simulink model "MagnetoShield_PolePlacement_UNO"  (R2019a)
settings: Solver=FixedStepAuto  StartTime=0.0  StopTime=10.0  RelTol=1e-3  EnableMultiTasking=on
undefined symbols (not defined in the file): A, B, C, DiscIntNeverNeededParam, i0, K, L, MEGA, Ts, u0, UNO, y0
libraries: MagnetoLibrary x2, CommonBlocks x1
settings Model: SimulationMode=external  ExtModeTrigDuration=2  Creator=jakub  LastModifiedBy=jakub
settings OptimizationCC: EnhancedBackFolding=on  PassReuseOutputArgsAs=Individual arguments  MaxStackSize=64  OptimizeBlockOrder=speed  DifferentSizesBufferReuse=on  OptimizationCustomize=off
settings DebuggingCC: ParameterTunabilityLossMsg=error
settings HardwareCC: ProdBitPerInt=16  ProdBitPerPointer=16  ProdBitPerSizeT=16  ProdBitPerPtrDiffT=16  ProdLargestAtomicFloat=None  ProdWordSize=8  ProdHWDeviceType=Atmel->AVR
settings SFSimCC: MATLABDynamicMemAlloc=off
settings RTWCC: SystemTargetFile=ert.tlc  HardwareBoard=Arduino Uno  TLCOptions=-aInlineSetEventsForThisBaseRateFcn=TLC_FALSE -aSuppressMultiTaskScheduler=TLC_FALSE -aRateBasedStepFcn=1  TemplateMakefile=ert_default_tmf  GenerateReport=on  Toolchain=Arduino AVR  BuildConfiguration=Faster Runs  IncludeHyperlinkInReport=on  LaunchReport=on  GenerateTraceInfo=on  GenerateTraceReport=on  GenerateTraceReportSl=on  GenerateTraceReportSf=on  GenerateTraceReportEml=on
settings CodeAppCC: ForceParamTrailComments=on  IgnoreCustomStorageClasses=off  OperatorAnnotations=on  SimulinkDataObjDesc=on  SFDataObjDesc=on  InsertBlockDesc=on
settings ERTTargetCC: SupportContinuousTime=on  SupportVariableSizeSignals=on  ExtModeStaticAllocSize=250

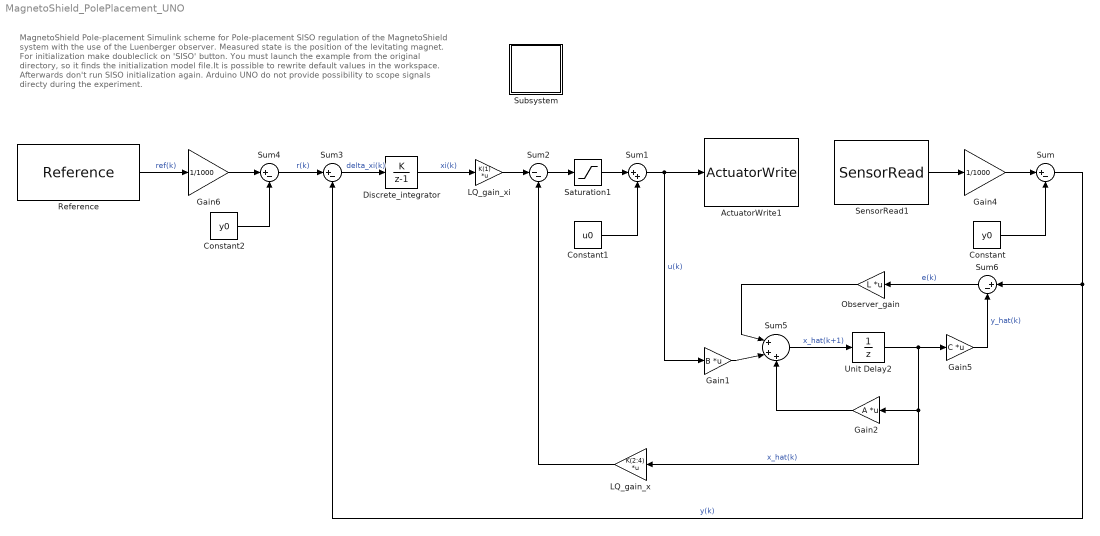
== system MagnetoShield_PolePlacement_UNO ==
  note: MagnetoShield Pole-placement
      | Simulink scheme for Pole-placement SISO regulation of the MagnetoShield system with the use of the Luenberger
      | observer. Measured state is the position of the levitating magnet.
      | For initialization make doubleclick on 'SISO' button. You must launch the example from the original directory, so it
      | finds the initialization model file.It is possible to rewrite default values in the workspace. Afterwards don't run SISO
      | initialization again.
      | Arduino UNO do not provide possibility to scope signals directy during the experiment.
  ActuatorWrite1 : MagnetoLibrary/ActuatorWrite  Board=UNO/MEGA  Units=Volts
      settings: SourceProductName=AutomationShield
  Constant : Constant  Value=y0
  Constant1 : Constant  Value=u0
  Constant2 : Constant  Value=y0
  Discrete_integrator : DiscreteIntegrator  IntegratorMethod=Accumulation: Forward Euler  SampleTime=Ts  LimitOutput=on  UpperSaturationLimit=1  LowerSaturationLimit=-1  ICPrevOutput=DiscIntNeverNeededParam  ICPrevScaledInput=DiscIntNeverNeededParam
  Gain1 : Gain  Gain=B  Multiplication=Matrix(K*u)
  Gain2 : Gain  Gain=A  Multiplication=Matrix(K*u)
  Gain4 : Gain  Gain=1/1000
  Gain5 : Gain  Gain=C  Multiplication=Matrix(K*u)
  Gain6 : Gain  Gain=1/1000
  LQ_gain_x : Gain  Gain=K(2:4)  Multiplication=Matrix(K*u)
  LQ_gain_xi : Gain  Gain=K(1)  Multiplication=Matrix(K*u)
  Observer_gain : Gain  Gain=L  Multiplication=Matrix(K*u)
  Reference : CommonBlocks/Reference  RefVect=[15, 13, 16, 14]  AtTheEnd=Start from beginning  Reps=5  SectLen=1000  OffsetTime=0  Ts=Ts
      settings: SourceProductName=AutomationShield
  Saturation1 : Saturate  UpperLimit=10-u0  LowerLimit=0-u0
  SensorRead1 : MagnetoLibrary/SensorRead  board=UNO/MEGA  sensor=Distance [mm]  sampling=Ts
      settings: SourceProductName=AutomationShield
  Subsystem : Subsystem
      settings: OpenFcn=|
      | clear;close all;clc;
      | cd(fileparts(which(gcs)));
      | load '../../../../matlab/examples/MagnetoShield/MagnetoShield_Models_Greybox_SS';
      | %% MagnetoShield - Pole-placement simulation and control initialization for Simulink
      | Ts = 0.0025;                   % Sampling of the Simulink simulation
      | 
      | % Matrices extraction from model
      | modeld=c2d(model,Ts);           % Discretized linear state-space model
      | A = modeld.a;                   % Extract A
      | B = modeld.b;                   % Extract B
      | C = [1 0 0];                   % Position is measured for integrator 'xi' computation
      | 
      | % Discrete augmented model with integrator state - unstable, unobservable
      | Ai = [1 -C;
      |       zeros(3,1) A];
      | Bi = [0;B];
      | 
      | % Observer gain L computation
      | polesL = [-0.003 0.0006715 -0.00003715]; % desired poles of observer
      | p = poly(polesL);                        % polynomial coeficients
      | I = eye(size(A));
      | phy = p(4)*I+p(3)*A+p(2)*A^2+A^3;
      | L = phy*inv([C; C*A; C*A^2])*[0 0 1]';   % Ackermann's formula for observer
      | 
      | % Pole-placement gain K for augmented system
      | polesK = [0.985 0.5353 0.826 0.9581];       % desired poles of the system
      | p = poly(polesK);                           % polynomial coeficients
      | I = eye(size(Ai));
      | phy = p(5)*I+p(4)*Ai+p(3)*Ai^2+p(2)*Ai^3+Ai^4;
      | K = [0 0 0 1]*inv([Bi Ai*Bi Ai^2*Bi Ai^3*Bi])*phy; % Ackermann's formula for gain K
      mask Display: disp('SISO')
  Sum{,3..4,6} (4 alike) : Sum  Inputs=|+-
  Sum1 : Sum  Inputs=|++
  Sum2 : Sum  Inputs=|--
  Sum5 : Sum  Inputs=|+++
  Unit Delay2 : UnitDelay  InitialCondition=[0.017-y0;0;0-i0]  SampleTime=-1  HasFrameUpgradeWarning=on
  wires:
  Constant2/1 -> Sum4/2
  LQ_gain_xi/1 -> Sum2/1
  Reference/1 -> Gain6/1  "ref(k)"
  Discrete_integrator/1 -> LQ_gain_xi/1  "xi(k)"
  Gain6/1 -> Sum4/1
  Gain1/1 -> Sum5/2
  Unit Delay2/1 -> Gain5/1, Gain2/1, LQ_gain_x/1  "x_hat(k)"
  LQ_gain_x/1 -> Sum2/2
  Saturation1/1 -> Sum1/1
  Sum/1 -> Sum6/1, Sum3/2  "y(k)"
  Sum4/1 -> Sum3/1  "r(k)"
  Sum6/1 -> Observer_gain/1  "e(k)"
  Gain5/1 -> Sum6/2  "y_hat(k)"
  Constant1/1 -> Sum1/2
  Sum1/1 -> ActuatorWrite1/1, Gain1/1  "u(k)"
  Constant/1 -> Sum/2
  Gain2/1 -> Sum5/3
  Sum5/1 -> Unit Delay2/1  "x_hat(k+1)"
  SensorRead1/1 -> Gain4/1
  Observer_gain/1 -> Sum5/1
  Sum2/1 -> Saturation1/1
  Sum3/1 -> Discrete_integrator/1  "delta_xi(k)"
  Gain4/1 -> Sum/1

== system MagnetoShield_PolePlacement_UNO/Subsystem ==
